simulink model "Demo919"  (R2018b)
settings: Solver=ode3  StartTime=0.0  StopTime=10  FixedStep=0.0005  RelTol=1e-3  EnableMultiTasking=on
values from neighbouring files (symbols this model uses):
  ADS1 = [1000 4000]    [data_new1.m]
  ADS2 = [900 4100]    [data_new1.m]
  br_opening = [0 20 40 60 80 100]    [data_new1.m]
  BRAKE = [485 1288 2091 2894 3697 4500]    [data_new1.m]
  InerWheel_Angle = [0 0.001 0.502 1.006 1.514 2.024 2.538 3.055 3.575 4.098 4.625 5.155 5.689 6.226 6.767 7.311 7.859 8.411 8.967 9.527 10.091 10.659 11.231 11.807 12.387 12.972 13.561 14.154 14.752 15.354 15.961 16.572 17.187 17.807 18.432 19.062 19.696 20.334 20.977 21.625 22.277 22.934 23.596 24.262 24.932 25.607 26.286 26.970 27.657 28.349 29.045 29.745 30.448 31.155 31.866]    [data_new1.m]
  OuterWheel_Angle = [0 0.001 0.501 1.001 1.501 2.001 2.501	3.001 3.501	4.001 4.501	5.001 5.501	6.001 6.501	7.001 7.501	8.001 8.501	9.001 9.501	10.001 10.501 11.001 11.501 12.001 12.501 13.001 13.501	14.001 14.501 15.001 15.501 16.001 16.501 17.001 17.501 18.001 18.501 19.001 19.501	20.001 20.501 21.001 21.501	22.001 22.501 23.001 23.501	24.001 24.501 25.001 25.501 26.001 26.501]    [data_new1.m]
  PUMP = [0 1000 2000 3000 4000 5000]    [data_new1.m]
  SteeringAngle_Cal = [-90 0 90]    [data_new1.m]
  SteeringAngle_Sensor = [640 1840 3041]    [data_new1.m]
  th_opening = [0 100]    [data_new1.m]
undefined symbols (not defined in the file or in its folder): D, I_AN06_5V, I_AN08_5V, I_AN09_5V, I_AN10_5V, I_HALL1, I_HALL2, I_SW01_L, I_SW10_L, I_SW11_H, I_SW12_H, I_SW13_H, I_SW14_H, I_SW15_H, I_SW16_H, I_SW17_H, I_SW18_H, I_SW19_H, I_SW20_H, O_PWM1_LS0A7, O_PWM2_LS0A7, O_SW02_LS0A4, O_SW13_HS1A, O_SW14_HS1A
libraries: ec5744lib x137, simulink x20, canmsglib x11
(part 3 of 5)

== system Demo919/Function-Call Subsystem1/Torque_Control/differential1 ==
  note: 转向半径计算模块
  note: 内外电机转速
  note: 转速差分配
  Steering_Angle : Inport
  Pedal_tr : Inport  Port=2
  MODE : Inport  Port=3
  Abs : Abs
  Add : Sum
  Constant1 : Constant  Value=10000
  Data Type Conversion : DataTypeConversion  OutDataTypeStr=double
  Data Type Conversion3 : DataTypeConversion  OutDataTypeStr=uint16
  Data Type Conversion4 : DataTypeConversion  OutDataTypeStr=uint16
  Gain3 : Gain  Gain=50
  Gain4 : Gain  Gain=2
  MeaModule1 : ec5744lib/RapidECU_U3/07Calibration/MeaModule  signal=InerMotor_RPM
      settings: SourceProductName=ECUCoder for MPC5744
  MeaModule3 : ec5744lib/RapidECU_U3/07Calibration/MeaModule  signal=OuterMotor_RPM
      settings: SourceProductName=ECUCoder for MPC5744
  RPM_Cal1 : Subsystem
  "SteeringAngle " : Subsystem
  Switch : Switch  Criteria=u2 > Threshold  Threshold=15
  Switch1 : Switch  Criteria=u2 > Threshold  Threshold=15
  dynamic_allocation : Stateflow chart  TreatAsAtomicUnit=on
  LMot_Speed : Outport
  RMot_Speed : Outport  Port=2
  SteeringAngle : Outport  Port=3
  wires:
  Steering_Angle/1 -> Data Type Conversion/1
  "SteeringAngle "/2(Turning radius) -> RPM_Cal1/3(Turning radius)
  "SteeringAngle "/1(LR_Flg) -> [LR_Flg]
  [LR_Flg] -> dynamic_allocation/1(LR_Flg)
  Data Type Conversion/1 -> "SteeringAngle "/1(sencor_data)
  RPM_Cal1/1(OuterMotor_RPM) -> MeaModule3/1
  RPM_Cal1/2(InerMotor_PRM) -> MeaModule1/1
  MeaModule3/1 -> Data Type Conversion3/1
  MeaModule1/1 -> Data Type Conversion4/1
  Data Type Conversion3/1 -> dynamic_allocation/2(OuterMotor_RPM)
  Data Type Conversion4/1 -> dynamic_allocation/3(InerMotor_RPM)
  MODE/1 -> RPM_Cal1/2("MODE ")
  Add/1 -> Gain4/1
  Pedal_tr/1 -> Gain3/1, RPM_Cal1/1(Pedal_tr)
  Gain4/1 -> Switch/3, Switch1/3
  "SteeringAngle "/3(SteeringAngle) -> Abs/1, SteeringAngle/1
  Gain3/1 -> Add/1
  Abs/1 -> Switch/2, Switch1/2
  Switch1/1 -> RMot_Speed/1
  Switch/1 -> LMot_Speed/1
  dynamic_allocation/1(LMot_Speed) -> Switch/1
  dynamic_allocation/2(RMot_Speed) -> Switch1/1
  Constant1/1 -> Add/2

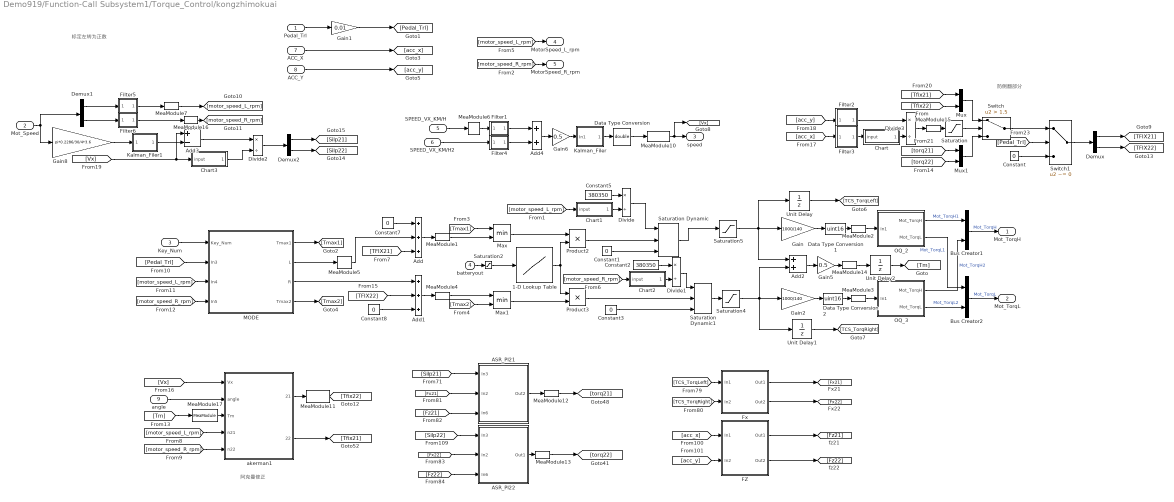
== system Demo919/Function-Call Subsystem1/Torque_Control/kongzhimokuai ==
  note: 阿克曼修正
  note: 防侧翻部分
  note: 标定左转为正数
  Pedal_Trl : Inport
  Mot_Speed : Inport  Port=2
  Key_Num : Inport  Port=3
  batteryout : Inport  Port=4
  SPEED_VX_KM/H : Inport  Port=5
  SPEED_VX_KM/H2 : Inport  Port=6
  ACC_X : Inport  Port=7
  ACC_Y : Inport  Port=8
  angle : Inport  Port=9
  1-D Lookup Table : Lookup_n-D  NumberOfTableDimensions=1  BreakpointsForDimension1=[0 10 20 30 40 50 60 70 72 74 76 78 80 85 100]  Table=[1 1 1 1 1 1 1 1 1 1 0.98 0.97 0.95 0.9 0.5]  InternalRulePriority=Speed  RndMeth=Simplest  InputSameDT=on
  ASR_PI21 : Subsystem
  ASR_PI22 : Subsystem
  Add : Sum  Inputs=+++
  Add1 : Sum  Inputs=+++
  Add2 : Sum
  Add3 : Sum  Inputs=+-
  Add4 : Sum
  Bus Creator1 : BusCreator  Inputs=2
  Bus Creator2 : BusCreator  Inputs=2
  Chart : Stateflow chart  TreatAsAtomicUnit=on
  Chart1 : Stateflow chart  TreatAsAtomicUnit=on
  Chart2 : Stateflow chart  TreatAsAtomicUnit=on
  Chart3 : Stateflow chart  TreatAsAtomicUnit=on
  Constant{,1,3,7..8} (5 alike) : Constant  Value=0
  Constant2 : Constant  Value=380350
  Constant5 : Constant  Value=380350
  Data Type Conversion : DataTypeConversion  OutDataTypeStr=double
  Data Type Conversion1 : DataTypeConversion  OutDataTypeStr=uint16  SaturateOnIntegerOverflow=on
  Data Type Conversion2 : DataTypeConversion  OutDataTypeStr=uint16  SaturateOnIntegerOverflow=on
  Demux : Demux  Outputs=2
  Demux1 : Demux  Outputs=2
  Demux2 : Demux  Outputs=2
  Divide{,1..3} (4 alike) : Product  Inputs=*/
  FZ : Subsystem
  Filter1 : Subsystem
  Filter2 : Subsystem
  Filter3 : Subsystem
  Filter4 : Subsystem
  Filter5 : Subsystem
  Filter6 : Subsystem
  Fx : Subsystem
  Gain : Gain  Gain=1000/140  OutDataTypeStr=double  SaturateOnIntegerOverflow=on
  Gain1 : Gain  Gain=0.01  OutDataTypeStr=double
  Gain2 : Gain  Gain=1000/140  OutDataTypeStr=double  SaturateOnIntegerOverflow=on
  Gain5 : Gain  Gain=0.5  OutDataTypeStr=double
  Gain6 : Gain  Gain=0.5  ParamDataTypeStr=single
  Gain8 : Gain  Gain=pi*0.2286/30/4*3.6
  Kalman_Filer : Subsystem
  Kalman_Filer1 : Subsystem
  MODE : Subsystem
  Max : MinMax  Inputs=2
  Max1 : MinMax  Inputs=2
  MeaModule1 : ec5744lib/RapidECU_U3/07Calibration/MeaModule  signal=c1
      settings: SourceProductName=ECUCoder for MPC5744
  MeaModule10 : ec5744lib/RapidECU_U3/07Calibration/MeaModule  signal=Speed
      settings: SourceProductName=ECUCoder for MPC5744
  MeaModule11 : ec5744lib/RapidECU_U3/07Calibration/MeaModule  signal=b9
      settings: SourceProductName=ECUCoder for MPC5744
  MeaModule12 : ec5744lib/RapidECU_U3/07Calibration/MeaModule  signal=c4
      settings: SourceProductName=ECUCoder for MPC5744
  MeaModule13 : ec5744lib/RapidECU_U3/07Calibration/MeaModule  signal=c5
      settings: SourceProductName=ECUCoder for MPC5744
  MeaModule14 : ec5744lib/RapidECU_U3/07Calibration/MeaModule  signal=c42
      settings: SourceProductName=ECUCoder for MPC5744
  MeaModule15 : ec5744lib/RapidECU_U3/07Calibration/MeaModule  signal=K
      settings: SourceProductName=ECUCoder for MPC5744
  MeaModule16 : ec5744lib/RapidECU_U3/07Calibration/MeaModule  signal=speed22
      settings: SourceProductName=ECUCoder for MPC5744
  MeaModule17 : ec5744lib/RapidECU_U3/07Calibration/MeaModule  signal=b7
      settings: SourceProductName=ECUCoder for MPC5744
  MeaModule2 : ec5744lib/RapidECU_U3/07Calibration/MeaModule  signal=C1
      settings: SourceProductName=ECUCoder for MPC5744
  MeaModule3 : ec5744lib/RapidECU_U3/07Calibration/MeaModule  signal=C2
      settings: SourceProductName=ECUCoder for MPC5744
  MeaModule4 : ec5744lib/RapidECU_U3/07Calibration/MeaModule  signal=c2
      settings: SourceProductName=ECUCoder for MPC5744
  MeaModule5 : ec5744lib/RapidECU_U3/07Calibration/MeaModule  signal=e1
      settings: SourceProductName=ECUCoder for MPC5744
  MeaModule6 : ec5744lib/RapidECU_U3/07Calibration/MeaModule  signal=S11
      settings: SourceProductName=ECUCoder for MPC5744
  MeaModule7 : ec5744lib/RapidECU_U3/07Calibration/MeaModule  signal=speed21
      settings: SourceProductName=ECUCoder for MPC5744
  Mux : Mux  Inputs=2
  Mux1 : Mux  Inputs=2
  OQ_2 : Subsystem
  OQ_3 : Subsystem
  Product2 : Product
  Product3 : Product
  Saturation : Saturate  UpperLimit=2.5  LowerLimit=-2.5
  Saturation Dynamic : simulink/Discontinuities/Saturation Dynamic  OutMin=[]  OutMax=[]  OutDataTypeStr=Inherit: Same as second input  OutDataType=fixdt(1, 16)  OutScaling=2^-10  DoSatur=on
  Saturation Dynamic1 : simulink/Discontinuities/Saturation Dynamic  OutMin=[]  OutMax=[]  OutDataTypeStr=Inherit: Same as second input  OutDataType=fixdt(1, 16)  OutScaling=2^-10  DoSatur=on
  Saturation2 : Saturate  UpperLimit=100  LowerLimit=0
  Saturation4 : Saturate  UpperLimit=140  LowerLimit=0
  Saturation5 : Saturate  UpperLimit=140  LowerLimit=0
  Switch : Switch  Criteria=u2 > Threshold  Threshold=1.5
  Switch1 : Switch  Criteria=u2 ~= 0
  Unit Delay : UnitDelay  SampleTime=-1
  Unit Delay1 : UnitDelay  SampleTime=-1
  Unit Delay2 : UnitDelay  SampleTime=-1
  akerman1 : Subsystem
  Mot_TorqH : Outport
  Mot_TorqL : Outport  Port=2
  speed : Outport  Port=3
  MotorSpeed_L_rpm : Outport  Port=4
  MotorSpeed_R_rpm : Outport  Port=5
  wires:
  [motor_speed_L_rpm] -> MotorSpeed_L_rpm/1
  [motor_speed_R_rpm] -> MotorSpeed_R_rpm/1
  Filter1/1(Out1) -> Add4/1
  Constant/1 -> Switch1/3
  Constant2/1 -> Divide1/1
  [TCS_TorqLeft] -> Fx/1(In1)
  [Vx] -> Chart3/1(input), Add3/1
  MeaModule2/1 -> OQ_2/1(In1)
  Unit Delay2/1 -> [Tm]
  Saturation/1 -> Switch/2
  Add3/1 -> Divide2/1
  Fx/1(Out1) -> [Fx21]
  Chart/1(output) -> Divide3/2
  MODE/1(Tmax1) -> [Tmax1]
  ACC_X/1 -> [acc_x]
  ASR_PI22/1(Out1) -> MeaModule13/1
  MODE/2(L) -> MeaModule5/1
  MeaModule12/1 -> [torq21]
  MeaModule14/1 -> Unit Delay2/1
  MODE/3(R) -> Add1/1
  FZ/1(Out1) -> [Fz21]
  [Silp22] -> ASR_PI22/1(In3)
  Kalman_Filer/1(Out1) -> Data Type Conversion/1
  Data Type Conversion1/1 -> MeaModule2/1
  Demux2/1 -> [Silp21]
  SPEED_VX_KM/H2/1 -> Filter4/1(In1)
  Demux/1 -> [TFIX21]
  Chart3/1(output) -> Divide2/2
  Gain6/1 -> Kalman_Filer/1(In1)
  Add/1 -> MeaModule1/1
  [Tfix22] -> Mux/2
  MeaModule15/1 -> Saturation/1
  [acc_y] -> FZ/2(In2)
  Add4/1 -> Gain6/1
  [Fx21] -> ASR_PI21/2(In2)
  Filter2/1(Out1) -> Divide3/1
  Unit Delay1/1 -> [TCS_TorqRight]
  Pedal_Trl/1 -> Gain1/1
  [acc_y] -> Filter2/1(In1)
  Constant1/1 -> Saturation Dynamic/3
  Filter3/1(Out1) -> Chart/1(input)
  Unit Delay/1 -> [TCS_TorqLeft]
  [motor_speed_L_rpm] -> Chart1/1(input)
  Bus Creator1/1 -> Mot_TorqH/1  "Mot_TorqH"
  MeaModule13/1 -> [torq22]
  Divide/1 -> Saturation Dynamic/1
  Demux2/2 -> [Silp22]
  FZ/2(Out2) -> [Fz22]
  Demux1/2 -> Filter6/1(In1)
  [motor_speed_L_rpm] -> MODE/3(In4)
  [Fz21] -> ASR_PI21/3(In6)
  [acc_x] -> Filter3/1(In1)
  SPEED_VX_KM/H/1 -> MeaModule6/1
  [motor_speed_R_rpm] -> Chart2/1(input)
  Demux/2 -> [TFIX22]
  Gain8/1 -> Kalman_Filer1/1(In1)
  Demux1/1 -> Filter5/1(In1)
  Mux/1 -> Switch/1
  Data Type Conversion2/1 -> MeaModule3/1
  OQ_2/1(Mot_TorqH) -> Bus Creator1/1  "Mot_TorqH1"
  [Fx22] -> ASR_PI22/2(In2)
  [Fz22] -> ASR_PI22/3(In6)
  Mux1/1 -> Switch/3
  [motor_speed_R_rpm] -> MODE/4(In5)
  Divide3/1 -> MeaModule15/1
  Add1/1 -> MeaModule4/1
  MODE/4(Tmax2) -> [Tmax2]
  [acc_x] -> FZ/1(In1)
  Divide2/1 -> Demux2/1
  Fx/2(Out2) -> [Fx22]
  Chart2/1(output) -> Divide1/2
  Chart1/1(output) -> Divide/2
  [TCS_TorqRight] -> Fx/2(In2)
  OQ_3/2(Mot_TorqL) -> Bus Creator2/2  "Mot_TorqL2"
  ACC_Y/1 -> [acc_y]
  [Pedal_Trl] -> Switch1/2
  [torq21] -> Mux1/1
  batteryout/1 -> Saturation2/1
  Max1/1 -> Product3/2
  [Pedal_Trl] -> MODE/2(In3)
  Add2/1 -> Gain5/1
  Switch/1 -> Switch1/1
  Divide1/1 -> Saturation Dynamic1/1
  Filter4/1(Out1) -> Add4/2
  Constant5/1 -> Divide/1
  [Silp21] -> ASR_PI21/1(In3)
  Key_Num/1 -> MODE/1(Key_Num)
  ASR_PI21/1(Out2) -> MeaModule12/1
  OQ_2/2(Mot_TorqL) -> Bus Creator2/1  "Mot_TorqL1"
  Bus Creator2/1 -> Mot_TorqL/1  "Mot_TorqL"
  Gain2/1 -> Data Type Conversion2/1
  Gain/1 -> Data Type Conversion1/1
  MeaModule3/1 -> OQ_3/1(In1)
  Max/1 -> Product2/1
  Gain5/1 -> MeaModule14/1
  [torq22] -> Mux1/2
  OQ_3/1(Mot_TorqH) -> Bus Creator1/2  "Mot_TorqH2"
  [Tfix21] -> Mux/1
  Switch1/1 -> Demux/1
  MeaModule5/1 -> Add/2
  Mot_Speed/1 -> Demux1/1, Gain8/1
  Gain1/1 -> [Pedal_Trl]
  [Tmax1] -> Max/1
  [Tmax2] -> Max1/2
  Data Type Conversion/1 -> MeaModule10/1
  MeaModule6/1 -> Filter1/1(In1)
  Kalman_Filer1/1(Out1) -> Add3/2
  Saturation2/1 -> 1-D Lookup Table/1
  MeaModule10/1 -> [Vx], speed/1
  Constant8/1 -> Add1/3
  Constant7/1 -> Add/1
  1-D Lookup Table/1 -> Product2/2, Product3/1
  Filter5/1(Out1) -> MeaModule7/1
  Filter6/1(Out1) -> MeaModule16/1
  MeaModule7/1 -> [motor_speed_L_rpm]
  MeaModule16/1 -> [motor_speed_R_rpm]
  Product2/1 -> Saturation Dynamic/2
  Saturation Dynamic/1 -> Saturation5/1
  Product3/1 -> Saturation Dynamic1/2
  Constant3/1 -> Saturation Dynamic1/3
  Saturation Dynamic1/1 -> Saturation4/1
  MeaModule11/1 -> [Tfix22]
  [motor_speed_R_rpm] -> akerman1/5(n22)
  angle/1 -> akerman1/2(angle)
  [Vx] -> akerman1/1("Vx ")
  akerman1/2("22 ") -> [Tfix21]
  MeaModule17/1 -> akerman1/3("Tm ")
  [Tm] -> MeaModule17/1
  [motor_speed_L_rpm] -> akerman1/4(n21)
  akerman1/1(21) -> MeaModule11/1
  [TFIX21] -> Add/3
  [TFIX22] -> Add1/2
  MeaModule1/1 -> Max/2
  MeaModule4/1 -> Max1/1
  Saturation5/1 -> Add2/1, Unit Delay/1, Gain/1
  Saturation4/1 -> Add2/2, Gain2/1, Unit Delay1/1

== system Demo919/Function-Call Subsystem1/Torque_Control/Subsystem1/Subsystem ==
  Pedal_WS1 : Inport
  Pedal_Ws2 : Inport  Port=2
  Pedal_Tr : Inport  Port=3
  Constant3 : Constant  Value=0  OutDataTypeStr=uint8
  Logical Operator : Logic  Operator=OR  AllPortsSameDT=off  OutDataTypeStr=boolean
  MeaModule9 : ec5744lib/RapidECU_U3/07Calibration/MeaModule  signal=Pedal_WrongState
      settings: SourceProductName=ECUCoder for MPC5744
  Pedal_Wo_Ar : Switch  Criteria=u2 > Threshold  OutDataTypeStr=double
  Out1 : Outport
  Pedal_WS : Outport  Port=2
  wires:
  MeaModule9/1 -> Pedal_Wo_Ar/2
  Pedal_Ws2/1 -> Logical Operator/2
  Constant3/1 -> Pedal_Wo_Ar/1
  Logical Operator/1 -> Pedal_WS/1, MeaModule9/1
  Pedal_WS1/1 -> Logical Operator/1
  Pedal_Tr/1 -> Pedal_Wo_Ar/3
  Pedal_Wo_Ar/1 -> Out1/1

== system Demo919/Function-Call Subsystem1/Torque_Control/differential1/RPM_Cal1 ==
  note: 计算期望转速和实际转速的误差输入pid，逐渐靠近期望
      | 在两个输出之后新增转速反馈pid
  note: 决定内外轮的速度差异
  note: 内外侧电机期望转速
  Pedal_tr : Inport
  "MODE " : Inport  Port=2
  Turning radius : Inport  Port=3
  Data Type Conversion : DataTypeConversion  OutDataTypeStr=double
  Divide2 : Product  Inputs=*/
  Divide3 : Product  Inputs=*/
  Divide6 : Product  Inputs=**
  Gain1 : Gain  Gain=60
  Gain2 : Gain  Gain=60
  Gain3 : Gain  Gain=4  OutDataTypeStr=double
  Gain4 : Gain  Gain=4  OutDataTypeStr=double
  Gain6 : Gain  Gain=1/100
  Gain7 : Gain  Gain=10/36
  Subsystem : Subsystem
  Tire_perimeter : Subsystem
  Tire_perimeter1 : Subsystem
  dynamic_allocation1 : Stateflow chart  TreatAsAtomicUnit=on
  OuterMotor_RPM : Outport  OutDataTypeStr=double
  InerMotor_PRM : Outport  Port=2  OutDataTypeStr=double
  wires:
  Divide2/1 -> Gain3/1
  Gain1/1 -> Divide2/1
  Gain2/1 -> Divide3/1
  Pedal_tr/1 -> Gain6/1
  Tire_perimeter1/1(D) -> Divide3/2
  Gain3/1 -> OuterMotor_RPM/1
  Divide3/1 -> Gain4/1
  Tire_perimeter/1(D) -> Divide2/2
  Gain4/1 -> InerMotor_PRM/1
  "MODE "/1 -> dynamic_allocation1/1(MODE)
  dynamic_allocation1/1(MAX_SPEED) -> Data Type Conversion/1
  Divide6/1 -> Subsystem/1(set_speed)
  Gain6/1 -> Divide6/2
  Gain7/1 -> Divide6/1
  Turning radius/1 -> Subsystem/2(Turning radius)
  Subsystem/1(Outer_speed) -> Gain1/1
  Subsystem/2(Iner_Speed) -> Gain2/1
  Data Type Conversion/1 -> Gain7/1

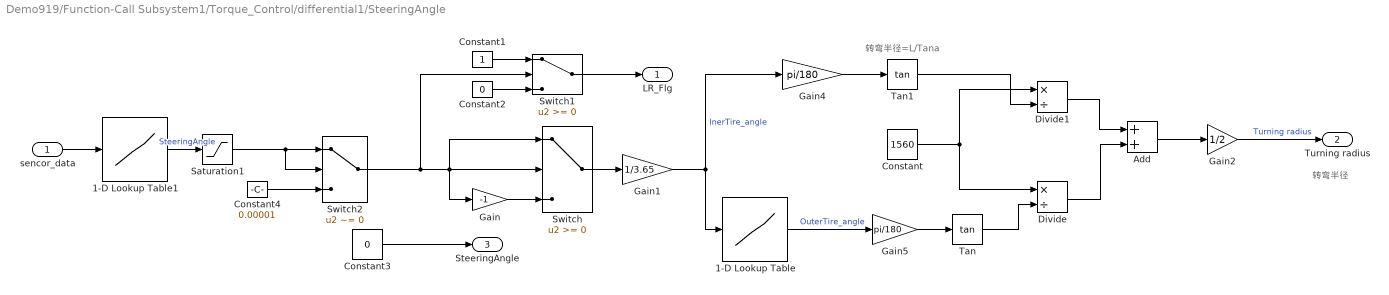
== system Demo919/Function-Call Subsystem1/Torque_Control/differential1/SteeringAngle  ==
  note: 转弯半径=L/Tana
  note: 转弯半径
  sencor_data : Inport
  1-D Lookup Table : Lookup_n-D  NumberOfTableDimensions=1  BreakpointsForDimension1=InerWheel_Angle  Table=OuterWheel_Angle  InternalRulePriority=Speed  RndMeth=Simplest  InputSameDT=on
  1-D Lookup Table1 : Lookup_n-D  NumberOfTableDimensions=1  BreakpointsForDimension1=SteeringAngle_Sensor  Table=SteeringAngle_Cal  InternalRulePriority=Speed  RndMeth=Simplest  InputSameDT=on
  Add : Sum
  Constant : Constant  Value=1560
  Constant1 : Constant
  Constant2 : Constant  Value=0
  Constant3 : Constant  Value=0
  Constant4 : Constant  Value=0.00001
  Divide : Product  Inputs=*/
  Divide1 : Product  Inputs=*/
  Gain : Gain  Gain=-1
  Gain1 : Gain  Gain=1/3.65
  Gain2 : Gain  Gain=1/2
  Gain4 : Gain  Gain=pi/180
  Gain5 : Gain  Gain=pi/180
  Saturation1 : Saturate  UpperLimit=90  LowerLimit=-90
  Switch : Switch
  Switch1 : Switch
  Switch2 : Switch  Criteria=u2 ~= 0
  Tan : Trigonometry  Operator=tan
  Tan1 : Trigonometry  Operator=tan
  LR_Flg : Outport
  Turning radius : Outport  Port=2
  SteeringAngle : Outport  Port=3
  wires:
  Gain1/1 -> Gain4/1, 1-D Lookup Table/1  "InerTire_angle"
  1-D Lookup Table/1 -> Gain5/1  "OuterTire_angle"
  1-D Lookup Table1/1 -> Saturation1/1  "SteeringAngle"
  Add/1 -> Gain2/1
  Divide/1 -> Add/2
  Gain/1 -> Switch/3
  Constant/1 -> Divide1/1, Divide/1
  Switch/1 -> Gain1/1
  Gain2/1 -> Turning radius/1  "Turning radius"
  Tan1/1 -> Divide1/2
  Tan/1 -> Divide/2
  Divide1/1 -> Add/1
  sencor_data/1 -> 1-D Lookup Table1/1
  Gain4/1 -> Tan1/1
  Gain5/1 -> Tan/1
  Constant1/1 -> Switch1/1
  Constant2/1 -> Switch1/3
  Switch1/1 -> LR_Flg/1
  Saturation1/1 -> Switch2/2, Switch2/1
  Constant4/1 -> Switch2/3
  Switch2/1 -> Switch/2, Switch/1, Gain/1, Switch1/2
  Constant3/1 -> SteeringAngle/1

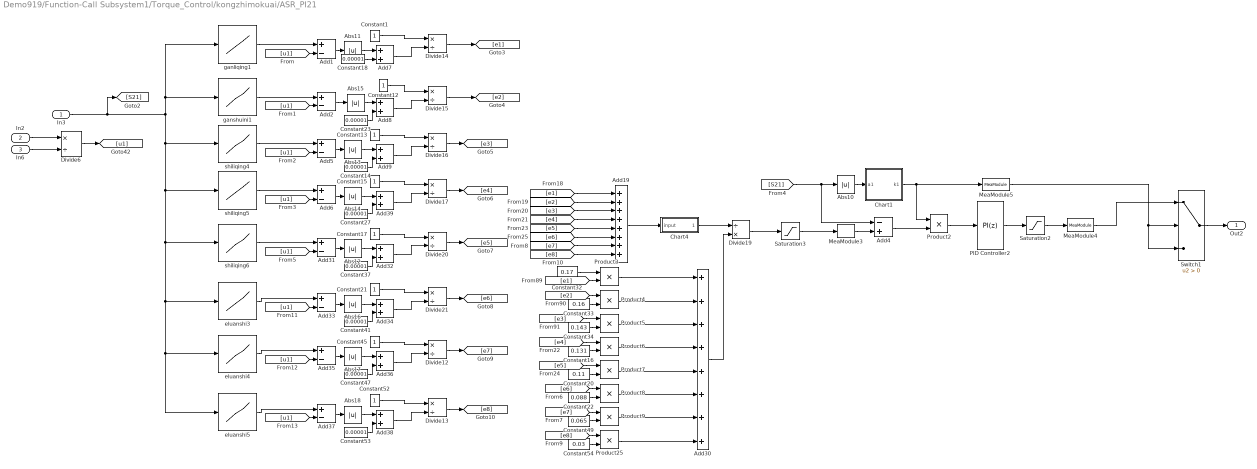
== system Demo919/Function-Call Subsystem1/Torque_Control/kongzhimokuai/ASR_PI21 ==
  In3 : Inport
  In2 : Inport  Port=2
  In6 : Inport  Port=3
  Abs{10..18} (9 alike) : Abs
  Add{1..2,5..6,31,33,35,37} (8 alike) : Sum  Inputs=+-
  Add19 : Sum  Inputs=++++++++
  Add30 : Sum  Inputs=++++++++
  Add{7..9,32,34,36,38..39} (8 alike) : Sum
  Add4 : Sum  Inputs=-+
  Chart1 : Stateflow chart  TreatAsAtomicUnit=on
  Chart4 : Stateflow chart  TreatAsAtomicUnit=on
  Constant{1,12..13,15,17,21,45,52} (8 alike) : Constant
  Constant{14,18,23,27,37,41,47,53} (8 alike) : Constant  Value=0.00001
  Constant16 : Constant  Value=0.131
  Constant20 : Constant  Value=0.11
  Constant22 : Constant  Value=0.088
  Constant32 : Constant  Value=0.17
  Constant33 : Constant  Value=0.16
  Constant34 : Constant  Value=0.143
  Constant49 : Constant  Value=0.065
  Constant54 : Constant  Value=0.03
  Divide{6,12..17,20..21} (9 alike) : Product  Inputs=*/
  Divide19 : Product  Inputs=/*
  MeaModule3 : ec5744lib/RapidECU_U3/07Calibration/MeaModule  signal=s_t
      settings: SourceProductName=ECUCoder for MPC5744
  MeaModule4 : ec5744lib/RapidECU_U3/07Calibration/MeaModule  signal=S_21
      settings: SourceProductName=ECUCoder for MPC5744
  MeaModule5 : ec5744lib/RapidECU_U3/07Calibration/MeaModule  signal=S_211
      settings: SourceProductName=ECUCoder for MPC5744
  PID Controller2 : simulink/Continuous/PID Controller  Controller=PI  Form=Parallel  TimeDomain=Discrete-time  SampleTime=-1  IntegratorMethod=Forward Euler  FilterMethod=Forward Euler  ControllerParametersSource=internal  P=156  I=25  D=D  UseFilter=on  N=100  TunerSelectOption=Transfer Function Based (PID Tuner App)  InitialConditionSource=internal  InitialConditionForIntegrator=0  InitialConditionForFilter=0  DifferentiatorICPrevScaledInput=0  ExternalReset=none  TrackingMode=off  Kt=1  LimitOutput=on  UpperSaturationLimit=inf  LowerSaturationLimit=-inf  LinearizeAsGain=on  AntiWindupMode=clamping  Kb=1  POutMin=[]  POutMax=[]  IOutMin=[]  IOutMax=[]  DOutMin=[]  DOutMax=[]  NOutMin=[]  NOutMax=[]  SumOutMin=[]  SumOutMax=[]  SaturationOutMin=[]  SaturationOutMax=[]  PParamMin=[]  PParamMax=[]  IParamMin=[]  IParamMax=[]  DParamMin=[]  DParamMax=[]  NParamMin=[]  NParamMax=[]  KbParamMin=[]  KbParamMax=[]  KtParamMin=[]  KtParamMax=[]  KbOutMin=[]  KbOutMax=[]  KtOutMin=[]  KtOutMax=[]  IntegratorOutMin=[]  IntegratorOutMax=[]  FilterOutMin=[]  FilterOutMax=[]  SumI1OutMin=[]  SumI1OutMax=[]  SumI2OutMin=[]  SumI2OutMax=[]  SumI3OutMin=[]  SumI3OutMax=[]  SumI4OutMin=[]  SumI4OutMax=[]  SumDOutMin=[]  SumDOutMax=[]  DifferentiatorOutMin=[]  DifferentiatorOutMax=[]  FilterDiffOutCoefMin=[]  FilterDiffOutCoefMax=[]  ReciprocalOutMin=[]  ReciprocalOutMax=[]  SumDenOutMin=[]  SumDenOutMax=[]  SumNumOutMin=[]  SumNumOutMax=[]  DivideOutMin=[]  DivideOutMax=[]  IntegratorContinuousStateAttributes=''  IntegratorStateMustResolveToSignalObject=off  IntegratorRTWStateStorageClass=Auto  FilterContinuousStateAttributes=''  FilterStateMustResolveToSignalObject=off  FilterRTWStateStorageClass=Auto  ParallelPVariant=InternalParameters  IdealPVariant=Disabled  IVariant=InternalParameters  DVariant=Disabled  IntegratorVariant=Discrete  SatVariant=Enabled  AWVariant=DiscClampingParallel  PCopyVariant=Disabled  TRVariant=Disabled  FdbkBlocksVariant=Forward  IdealPFdbkVariant=Disabled  SatFdbkVariant=Disabled  DerivativeFilterVariant=Disabled  NVariant=Disabled  NCopyVariant=Disabled_SignalSpec  FilterICVariant=Disabled  IntegratorICVariant=InternalICs  ExternalResetVariant=Disabled  TRSumVariant=Passthrough  SumFdbkVariant=Disabled  SumVariant=Sum_PI
  Product{2..9,25} (9 alike) : Product
  Saturation2 : Saturate  UpperLimit=15  LowerLimit=-15
  Saturation3 : Saturate  UpperLimit=0.2  LowerLimit=0
  Switch1 : Switch  Criteria=u2 > Threshold
  eluanshi3 : Lookup_n-D  NumberOfTableDimensions=1  BreakpointsForDimension1=[0.00591,0.009,0.01212,0.01856,0.0196,0.02707,0.03557,0.04385,0.05236,0.06524,0.1011,0.13927,0.18595,0.21975,0.26849,0.32574,0.38507,0.44646,0.51635,0.58188,0.63914,0.70697,0.78123,0.86792,0.92103,0.97184,0.993]  Table=[0.04929,0.12757,0.19671,0.25086,0.2838,0.31087,0.34088,0.36501,0.38001,0.38915,0.38915,0.38621,0.38295,0.37414,0.37121,0.36208,0.35588,0.34707,0.33794,0.335,0.32587,0.31707,0.31087,0.2988,0.29293,0.28673,0.2838]  InternalRulePriority=Speed  RndMeth=Simplest  InputSameDT=on
  eluanshi4 : Lookup_n-D  NumberOfTableDimensions=1  BreakpointsForDimension1=|  Table=|  InternalRulePriority=Speed  RndMeth=Simplest  InputSameDT=on
      BreakpointsForDimension1=|
      | [0.00154
      | 0.00798
      | 0.01649
      | 0.0227
      | 0.03121
      | 0.04178
      | 0.05673
      | 0.12433
      | 0.19216
      | 0.26642
      | 0.36598
      | 0.4952
      | 0.61591
      | 0.79388
      | 0.91873
      | 1.00357]
      Table=|
      | [0.04636
      | 0.11257
      | 0.14257
      | 0.17551
      | 0.18465
      | 0.19052
      | 0.19052
      | 0.18758
      | 0.18465
      | 0.17551
      | 0.17258
      | 0.16051
      | 0.15758
      | 0.14551
      | 0.13638
      | 0.1305]
  eluanshi5 : Lookup_n-D  NumberOfTableDimensions=1  BreakpointsForDimension1=|  Table=|  InternalRulePriority=Speed  RndMeth=Simplest  InputSameDT=on
      BreakpointsForDimension1=|
      | [0.00361
      | 0.00798
      | 0.01212
      | 0.01419
      | 0.01856
      | 0.0227
      | 0.02707
      | 0.02914
      | 0.04178
      | 0.09903
      | 0.15836
      | 0.26435
      | 0.37012
      | 0.49934
      | 0.60327
      | 0.69225
      | 0.78537
      | 0.86792
      | 0.94425
      | 1.0015]
      Table=|
      | [0.05549
      | 0.1093
      | 0.13964
      | 0.1517
      | 0.16051
      | 0.16964
      | 0.17845
      | 0.18465
      | 0.19052
      | 0.19052
      | 0.18465
      | 0.17845
      | 0.17258
      | 0.16671
      | 0.15758
      | 0.15464
      | 0.14551
      | 0.14257
      | 0.13638
      | 0.13344]
  ganliqing1 : Lookup_n-D  NumberOfTableDimensions=1  BreakpointsForDimension1=|  Table=|  InternalRulePriority=Speed  RndMeth=Simplest  InputSameDT=on
      BreakpointsForDimension1=|
      | [0.01498
      | 0.03128
      | 0.05446
      | 0.06846
      | 0.08017
      | 0.09165
      | 0.10335
      | 0.11506
      | 0.12424
      | 0.13595
      | 0.15454
      | 0.16625
      | 0.17772
      | 0.19632
      | 0.22202
      | 0.25691
      | 0.31499
      | 0.38017
      | 0.49196
      | 0.59433
      | 0.70129
      | 0.80367
      | 0.86885
      | 0.95493
      | 0.999]
      Table=|
      | [0.38854
      | 0.66554
      | 0.92268
      | 1.00503
      | 1.04474
      | 1.08738
      | 1.12058
      | 1.13686
      | 1.1502
      | 1.16322
      | 1.1668
      | 1.1668
      | 1.1668
      | 1.16322
      | 1.15346
      | 1.14044
      | 1.11049
      | 1.07762
      | 1.02489
      | 0.9689
      | 0.91617
      | 0.86019
      | 0.82699
      | 0.78435
      | 0.76123]
  ganshuini1 : Lookup_n-D  NumberOfTableDimensions=1  BreakpointsForDimension1=|  Table=|  InternalRulePriority=Speed  RndMeth=Simplest  InputSameDT=on
      BreakpointsForDimension1=|
      | [0
      | 0.00612
      | 0.01323
      | 0.0185
      | 0.024
      | 0.03293
      | 0.04531
      | 0.05241
      | 0.06295
      | 0.06845
      | 0.07555
      | 0.08266
      | 0.08976
      | 0.0932
      | 0.10213
      | 0.11107
      | 0.12161
      | 0.13055
      | 0.14315
      | 0.15369
      | 0.17156
      | 0.18577
      | 0.19631
      | 0.21419
      | 0.2355
      | 0.25497
      | 0.27468
      | 0.28889
      | 0.30676
      | 0.3173
      | 0.33334
      | 0.35465
      | 0.37252
      | 0.3991
      | 0.41858
      | 0.44539
      | 0.46143
      | 0.48985
      | 0.51299
      | 0.53613
      | 0.55194
      | 0.56798
      | 0.59823
      | 0.6161
      | 0.64085
      | 0.66926
      | 0.69424
      | 0.69791
      | 0.71211
      | 0.75107
      | 0.79209
      | 0.81706
      | 0.85075
      | 0.89887
      | 0.93599
      | 0.98411
      | 0.99832]
      Table=|
      | [0.0357
      | 0.13134
      | 0.30251
      | 0.41079
      | 0.52393
      | 0.63999
      | 0.78847
      | 0.84617
      | 0.90679
      | 0.9444
      | 0.97228
      | 0.99238
      | 1.01248
      | 1.02512
      | 1.04263
      | 1.05787
      | 1.06532
      | 1.07537
      | 1.07797
      | 1.08056
      | 1.08056
      | 1.07797
      | 1.07537
      | 1.06792
      | 1.05527
      | 1.05009
      | 1.04004
      | 1.03258
      | 1.02512
      | 1.01994
      | 1.00989
      | 0.99724
      | 0.98979
      | 0.97455
      | 0.9645
      | 0.94959
      | 0.94181
      | 0.92949
      | 0.91425
      | 0.90161
      | 0.89156
      | 0.8841
      | 0.86886
      | 0.86141
      | 0.84876
      | 0.82867
      | 0.81602
      | 0.81343
      | 0.80857
      | 0.78587
      | 0.76318
      | 0.75313
      | 0.73562
      | 0.70547
      | 0.69024
      | 0.66268
      | 0.6549]
  shiliqing4 : Lookup_n-D  NumberOfTableDimensions=1  BreakpointsForDimension1=|  Table=|  InternalRulePriority=Speed  RndMeth=Simplest  InputSameDT=on
      BreakpointsForDimension1=|
      | [0.00269
      | 0.00429
      | 0.01139
      | 0.01689
      | 0.02033
      | 0.0256
      | 0.0311
      | 0.04004
      | 0.04874
      | 0.06135
      | 0.07372
      | 0.08609
      | 0.0987
      | 0.11451
      | 0.13948
      | 0.1734
      | 0.20342
      | 0.23023
      | 0.24787
      | 0.26391
      | 0.28522
      | 0.30676
      | 0.3173
      | 0.35465
      | 0.39383
      | 0.42935
      | 0.47564
      | 0.51826
      | 0.55905
      | 0.59113
      | 0.63925
      | 0.68003
      | 0.72266
      | 0.7529
      | 0.79552
      | 0.84548
      | 0.89153
      | 0.92545
      | 0.99488]
      Table=|
      | [0.04835
      | 0.16927
      | 0.24707
      | 0.3278
      | 0.39328
      | 0.54662
      | 0.63221
      | 0.70547
      | 0.76059
      | 0.82607
      | 0.87405
      | 0.89901
      | 0.9243
      | 0.93694
      | 0.93954
      | 0.93694
      | 0.92689
      | 0.92171
      | 0.90906
      | 0.9042
      | 0.89415
      | 0.8841
      | 0.87665
      | 0.864
      | 0.84876
      | 0.82867
      | 0.81116
      | 0.79592
      | 0.77323
      | 0.75832
      | 0.74049
      | 0.72298
      | 0.70029
      | 0.69024
      | 0.67014
      | 0.64744
      | 0.62994
      | 0.6147
      | 0.58196]
  shiliqing5 : Lookup_n-D  NumberOfTableDimensions=1  BreakpointsForDimension1=|  Table=|  InternalRulePriority=Speed  RndMeth=Simplest  InputSameDT=on
      BreakpointsForDimension1=|
      | [8.52288E-4
      | 0.00429
      | 0.00612
      | 0.00796
      | 0.01139
      | 0.01506
      | 0.01689
      | 0.0185
      | 0.02033
      | 0.02216
      | 0.0256
      | 0.02927
      | 0.03454
      | 0.0382
      | 0.04164
      | 0.04714
      | 0.05058
      | 0.05768
      | 0.06478
      | 0.07189
      | 0.08082
      | 0.08793
      | 0.0932
      | 0.0987
      | 0.1058
      | 0.1129
      | 0.12528
      | 0.14315
      | 0.1876
      | 0.21052
      | 0.23023
      | 0.25337
      | 0.29072
      | 0.33678
      | 0.40437
      | 0.48435
      | 0.55561
      | 0.6035
      | 0.70662
      | 0.76894
      | 0.84364
      | 0.92018
      | 1.00015]
      Table=|
      | [0.04575
      | 0.09859
      | 0.14139
      | 0.19423
      | 0.24221
      | 0.285
      | 0.33525
      | 0.37059
      | 0.40074
      | 0.43348
      | 0.46622
      | 0.53171
      | 0.56672
      | 0.59201
      | 0.62475
      | 0.65231
      | 0.675
      | 0.71034
      | 0.73789
      | 0.75313
      | 0.77064
      | 0.77842
      | 0.78328
      | 0.78847
      | 0.79592
      | 0.79852
      | 0.79852
      | 0.79333
      | 0.78587
      | 0.77842
      | 0.77064
      | 0.76577
      | 0.75313
      | 0.73562
      | 0.71293
      | 0.68505
      | 0.66009
      | 0.64485
      | 0.6147
      | 0.58715
      | 0.56186
      | 0.53657
      | 0.50902]
  shiliqing6 : Lookup_n-D  NumberOfTableDimensions=1  BreakpointsForDimension1=|  Table=|  InternalRulePriority=Speed  RndMeth=Simplest  InputSameDT=on
      BreakpointsForDimension1=|
      | [0.0
      | 0.00154
      | 0.00798
      | 0.01212
      | 0.01419
      | 0.01856
      | 0.02477
      | 0.02914
      | 0.03764
      | 0.04615
      | 0.05236
      | 0.05673
      | 0.06087
      | 0.06937
      | 0.07788
      | 0.08846
      | 0.10317
      | 0.11812
      | 0.1372
      | 0.16893
      | 0.20503
      | 0.24941
      | 0.29171
      | 0.32988
      | 0.37012
      | 0.41243
      | 0.45496
      | 0.49083
      | 0.529
      | 0.57775
      | 0.62856
      | 0.68167
      | 0.73249
      | 0.77686
      | 0.82975
      | 0.90608
      | 0.94839
      | 1]
      Table=|
      | [0.0
      | 0.09756
      | 0.14551
      | 0.20878
      | 0.25379
      | 0.32
      | 0.35588
      | 0.39208
      | 0.44329
      | 0.47917
      | 0.50624
      | 0.5245
      | 0.5395
      | 0.55451
      | 0.57245
      | 0.58158
      | 0.59071
      | 0.59952
      | 0.59658
      | 0.59365
      | 0.58745
      | 0.57864
      | 0.57245
      | 0.56364
      | 0.55451
      | 0.54831
      | 0.5395
      | 0.53331
      | 0.5245
      | 0.51537
      | 0.5033
      | 0.49417
      | 0.48536
      | 0.47623
      | 0.46416
      | 0.44916
      | 0.44329
      | 0.43122]
  Out2 : Outport
  wires:
  MeaModule3/1 -> Add4/2
  Add4/1 -> Product2/2
  PID Controller2/1 -> Saturation2/1
  Add19/1 -> Chart4/1(input)
  Constant13/1 -> Divide16/1
  MeaModule4/1 -> Switch1/1
  In2/1 -> Divide6/1
  Divide6/1 -> [u1]
  Chart1/1(k1) -> Product2/1, MeaModule5/1
  [S21] -> Abs10/1, Add4/1
  In3/1 -> [S21], ganliqing1/1, ganshuini1/1, eluanshi4/1, eluanshi5/1, eluanshi3/1, shiliqing6/1, shiliqing5/1, shiliqing4/1
  Add33/1 -> Abs16/1
  Add39/1 -> Divide17/2
  Add35/1 -> Abs17/1
  Constant22/1 -> Product8/2
  eluanshi5/1 -> Add37/1
  [e7] -> Product9/1
  Constant54/1 -> Product25/2
  Constant27/1 -> Add39/2
  Constant21/1 -> Divide21/1
  Constant34/1 -> Product5/2
  Product4/1 -> Add30/2
  Constant33/1 -> Product4/2
  Divide15/1 -> [e2]
  Abs12/1 -> Add32/1
  Constant16/1 -> Product6/2
  Constant47/1 -> Add36/2
  shiliqing4/1 -> Add5/1
  Add37/1 -> Abs18/1
  eluanshi3/1 -> Add33/1
  [e5] -> Add19/5
  [e4] -> Product6/1
  Add8/1 -> Divide15/2
  Constant15/1 -> Divide17/1
  Add9/1 -> Divide16/2
  [e6] -> Product8/1
  Constant23/1 -> Add8/2
  [e1] -> Add19/1
  Add6/1 -> Abs14/1
  [e2] -> Add19/2
  Add7/1 -> Divide14/2
  Constant32/1 -> Product3/1
  Abs15/1 -> Add8/1
  Saturation3/1 -> MeaModule3/1
  [u1] -> Add6/2
  [u1] -> Add31/2
  Abs14/1 -> Add39/1
  Divide13/1 -> [e8]
  [u1] -> Add37/2
  Abs13/1 -> Add9/1
  Abs17/1 -> Add36/1
  Abs18/1 -> Add38/1
  Abs16/1 -> Add34/1
  [e7] -> Add19/7
  Add5/1 -> Abs13/1
  ganshuini1/1 -> Add2/1
  Divide20/1 -> [e5]
  Add38/1 -> Divide13/2
  Divide17/1 -> [e4]
  [u1] -> Add5/2
  Constant45/1 -> Divide12/1
  Add34/1 -> Divide21/2
  [u1] -> Add1/2
  Divide14/1 -> [e1]
  Constant53/1 -> Add38/2
  [e8] -> Product25/1
  Constant17/1 -> Divide20/1
  shiliqing6/1 -> Add31/1
  Product9/1 -> Add30/7
  Divide21/1 -> [e6]
  Product25/1 -> Add30/8
  Add1/1 -> Abs11/1
  [e8] -> Add19/8
  [e3] -> Product5/1
  Product5/1 -> Add30/3
  shiliqing5/1 -> Add6/1
  [e5] -> Product7/1
  [e3] -> Add19/3
  Constant12/1 -> Divide15/1
  Abs10/1 -> Chart1/1(a1)
  Product2/1 -> PID Controller2/1
  Constant14/1 -> Add9/2
  ganliqing1/1 -> Add1/1
  [u1] -> Add33/2
  Saturation2/1 -> MeaModule4/1
  Constant20/1 -> Product7/2
  Add31/1 -> Abs12/1
  Add2/1 -> Abs15/1
  Constant37/1 -> Add32/2
  Switch1/1 -> Out2/1
  Divide19/1 -> Saturation3/1
  [e4] -> Add19/4
  Product8/1 -> Add30/6
  Product3/1 -> Add30/1
  Constant18/1 -> Add7/2
  Add30/1 -> Divide19/2
  Divide16/1 -> [e3]
  [e2] -> Product4/1
  eluanshi4/1 -> Add35/1
  Constant41/1 -> Add34/2
  [e6] -> Add19/6
  [u1] -> Add2/2
  In6/1 -> Divide6/2
  Constant1/1 -> Divide14/1
  Product6/1 -> Add30/4
  [u1] -> Add35/2
  [e1] -> Product3/2
  MeaModule5/1 -> Switch1/3, Switch1/2
  Constant52/1 -> Divide13/1
  Constant49/1 -> Product9/2
  Add32/1 -> Divide20/2
  Divide12/1 -> [e7]
  Chart4/1(output) -> Divide19/1
  Add36/1 -> Divide12/2
  Product7/1 -> Add30/5
  Abs11/1 -> Add7/1

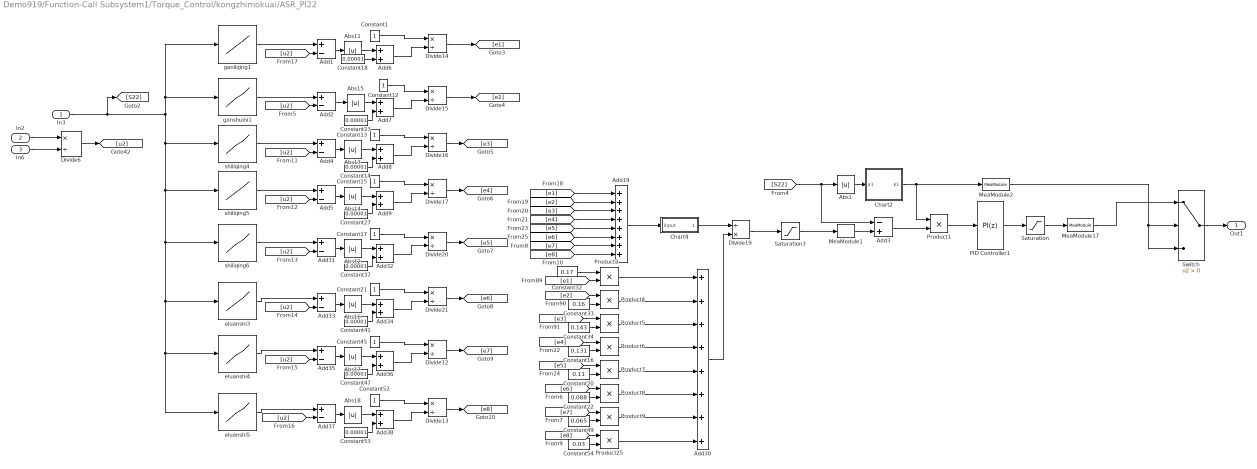
== system Demo919/Function-Call Subsystem1/Torque_Control/kongzhimokuai/ASR_PI22 ==
  In3 : Inport
  In2 : Inport  Port=2
  In6 : Inport  Port=3
  Abs{1,11..18} (9 alike) : Abs
  Add{1..2,4..5,31,33,35,37} (8 alike) : Sum  Inputs=+-
  Add19 : Sum  Inputs=++++++++
  Add3 : Sum  Inputs=-+
  Add30 : Sum  Inputs=++++++++
  Add{6..9,32,34,36,38} (8 alike) : Sum
  Chart2 : Stateflow chart  TreatAsAtomicUnit=on
  Chart4 : Stateflow chart  TreatAsAtomicUnit=on
  Constant{1,12..13,15,17,21,45,52} (8 alike) : Constant
  Constant{14,18,23,27,37,41,47,53} (8 alike) : Constant  Value=0.00001
  Constant16 : Constant  Value=0.131
  Constant20 : Constant  Value=0.11
  Constant22 : Constant  Value=0.088
  Constant32 : Constant  Value=0.17
  Constant33 : Constant  Value=0.16
  Constant34 : Constant  Value=0.143
  Constant49 : Constant  Value=0.065
  Constant54 : Constant  Value=0.03
  Divide{6,12..17,20..21} (9 alike) : Product  Inputs=*/
  Divide19 : Product  Inputs=/*
  MeaModule1 : ec5744lib/RapidECU_U3/07Calibration/MeaModule  signal=s_t7
      settings: SourceProductName=ECUCoder for MPC5744
  MeaModule17 : ec5744lib/RapidECU_U3/07Calibration/MeaModule  signal=S_217
      settings: SourceProductName=ECUCoder for MPC5744
  MeaModule2 : ec5744lib/RapidECU_U3/07Calibration/MeaModule  signal=S_2117
      settings: SourceProductName=ECUCoder for MPC5744
  PID Controller1 : simulink/Continuous/PID Controller  Controller=PI  Form=Parallel  TimeDomain=Discrete-time  SampleTime=-1  IntegratorMethod=Forward Euler  FilterMethod=Forward Euler  ControllerParametersSource=internal  P=156  I=25  D=D  UseFilter=on  N=100  TunerSelectOption=Transfer Function Based (PID Tuner App)  InitialConditionSource=internal  InitialConditionForIntegrator=0  InitialConditionForFilter=0  DifferentiatorICPrevScaledInput=0  ExternalReset=none  TrackingMode=off  Kt=1  LimitOutput=on  UpperSaturationLimit=inf  LowerSaturationLimit=-inf  LinearizeAsGain=on  AntiWindupMode=clamping  Kb=1  POutMin=[]  POutMax=[]  IOutMin=[]  IOutMax=[]  DOutMin=[]  DOutMax=[]  NOutMin=[]  NOutMax=[]  SumOutMin=[]  SumOutMax=[]  SaturationOutMin=[]  SaturationOutMax=[]  PParamMin=[]  PParamMax=[]  IParamMin=[]  IParamMax=[]  DParamMin=[]  DParamMax=[]  NParamMin=[]  NParamMax=[]  KbParamMin=[]  KbParamMax=[]  KtParamMin=[]  KtParamMax=[]  KbOutMin=[]  KbOutMax=[]  KtOutMin=[]  KtOutMax=[]  IntegratorOutMin=[]  IntegratorOutMax=[]  FilterOutMin=[]  FilterOutMax=[]  SumI1OutMin=[]  SumI1OutMax=[]  SumI2OutMin=[]  SumI2OutMax=[]  SumI3OutMin=[]  SumI3OutMax=[]  SumI4OutMin=[]  SumI4OutMax=[]  SumDOutMin=[]  SumDOutMax=[]  DifferentiatorOutMin=[]  DifferentiatorOutMax=[]  FilterDiffOutCoefMin=[]  FilterDiffOutCoefMax=[]  ReciprocalOutMin=[]  ReciprocalOutMax=[]  SumDenOutMin=[]  SumDenOutMax=[]  SumNumOutMin=[]  SumNumOutMax=[]  DivideOutMin=[]  DivideOutMax=[]  IntegratorContinuousStateAttributes=''  IntegratorStateMustResolveToSignalObject=off  IntegratorRTWStateStorageClass=Auto  FilterContinuousStateAttributes=''  FilterStateMustResolveToSignalObject=off  FilterRTWStateStorageClass=Auto  ParallelPVariant=InternalParameters  IdealPVariant=Disabled  IVariant=InternalParameters  DVariant=Disabled  IntegratorVariant=Discrete  SatVariant=Enabled  AWVariant=DiscClampingParallel  PCopyVariant=Disabled  TRVariant=Disabled  FdbkBlocksVariant=Forward  IdealPFdbkVariant=Disabled  SatFdbkVariant=Disabled  DerivativeFilterVariant=Disabled  NVariant=Disabled  NCopyVariant=Disabled_SignalSpec  FilterICVariant=Disabled  IntegratorICVariant=InternalICs  ExternalResetVariant=Disabled  TRSumVariant=Passthrough  SumFdbkVariant=Disabled  SumVariant=Sum_PI
  Product{1,3..9,25} (9 alike) : Product
  Saturation : Saturate  UpperLimit=15  LowerLimit=-15
  Saturation3 : Saturate  UpperLimit=0.2  LowerLimit=0
  Switch : Switch  Criteria=u2 > Threshold
  eluanshi3 : Lookup_n-D  NumberOfTableDimensions=1  BreakpointsForDimension1=[0.00591,0.009,0.01212,0.01856,0.0196,0.02707,0.03557,0.04385,0.05236,0.06524,0.1011,0.13927,0.18595,0.21975,0.26849,0.32574,0.38507,0.44646,0.51635,0.58188,0.63914,0.70697,0.78123,0.86792,0.92103,0.97184,0.993]  Table=[0.04929,0.12757,0.19671,0.25086,0.2838,0.31087,0.34088,0.36501,0.38001,0.38915,0.38915,0.38621,0.38295,0.37414,0.37121,0.36208,0.35588,0.34707,0.33794,0.335,0.32587,0.31707,0.31087,0.2988,0.29293,0.28673,0.2838]  InternalRulePriority=Speed  RndMeth=Simplest  InputSameDT=on
  eluanshi4 : Lookup_n-D  NumberOfTableDimensions=1  BreakpointsForDimension1=|  Table=|  InternalRulePriority=Speed  RndMeth=Simplest  InputSameDT=on
      BreakpointsForDimension1=|
      | [0.00154
      | 0.00798
      | 0.01649
      | 0.0227
      | 0.03121
      | 0.04178
      | 0.05673
      | 0.12433
      | 0.19216
      | 0.26642
      | 0.36598
      | 0.4952
      | 0.61591
      | 0.79388
      | 0.91873
      | 1.00357]
      Table=|
      | [0.04636
      | 0.11257
      | 0.14257
      | 0.17551
      | 0.18465
      | 0.19052
      | 0.19052
      | 0.18758
      | 0.18465
      | 0.17551
      | 0.17258
      | 0.16051
      | 0.15758
      | 0.14551
      | 0.13638
      | 0.1305]
  eluanshi5 : Lookup_n-D  NumberOfTableDimensions=1  BreakpointsForDimension1=|  Table=|  InternalRulePriority=Speed  RndMeth=Simplest  InputSameDT=on
      BreakpointsForDimension1=|
      | [0.00361
      | 0.00798
      | 0.01212
      | 0.01419
      | 0.01856
      | 0.0227
      | 0.02707
      | 0.02914
      | 0.04178
      | 0.09903
      | 0.15836
      | 0.26435
      | 0.37012
      | 0.49934
      | 0.60327
      | 0.69225
      | 0.78537
      | 0.86792
      | 0.94425
      | 1.0015]
      Table=|
      | [0.05549
      | 0.1093
      | 0.13964
      | 0.1517
      | 0.16051
      | 0.16964
      | 0.17845
      | 0.18465
      | 0.19052
      | 0.19052
      | 0.18465
      | 0.17845
      | 0.17258
      | 0.16671
      | 0.15758
      | 0.15464
      | 0.14551
      | 0.14257
      | 0.13638
      | 0.13344]
  ganliqing1 : Lookup_n-D  NumberOfTableDimensions=1  BreakpointsForDimension1=|  Table=|  InternalRulePriority=Speed  RndMeth=Simplest  InputSameDT=on
      BreakpointsForDimension1=|
      | [0.01498
      | 0.03128
      | 0.05446
      | 0.06846
      | 0.08017
      | 0.09165
      | 0.10335
      | 0.11506
      | 0.12424
      | 0.13595
      | 0.15454
      | 0.16625
      | 0.17772
      | 0.19632
      | 0.22202
      | 0.25691
      | 0.31499
      | 0.38017
      | 0.49196
      | 0.59433
      | 0.70129
      | 0.80367
      | 0.86885
      | 0.95493
      | 0.999]
      Table=|
      | [0.38854
      | 0.66554
      | 0.92268
      | 1.00503
      | 1.04474
      | 1.08738
      | 1.12058
      | 1.13686
      | 1.1502
      | 1.16322
      | 1.1668
      | 1.1668
      | 1.1668
      | 1.16322
      | 1.15346
      | 1.14044
      | 1.11049
      | 1.07762
      | 1.02489
      | 0.9689
      | 0.91617
      | 0.86019
      | 0.82699
      | 0.78435
      | 0.76123]
  ganshuini1 : Lookup_n-D  NumberOfTableDimensions=1  BreakpointsForDimension1=|  Table=|  InternalRulePriority=Speed  RndMeth=Simplest  InputSameDT=on
      BreakpointsForDimension1=|
      | [0
      | 0.00612
      | 0.01323
      | 0.0185
      | 0.024
      | 0.03293
      | 0.04531
      | 0.05241
      | 0.06295
      | 0.06845
      | 0.07555
      | 0.08266
      | 0.08976
      | 0.0932
      | 0.10213
      | 0.11107
      | 0.12161
      | 0.13055
      | 0.14315
      | 0.15369
      | 0.17156
      | 0.18577
      | 0.19631
      | 0.21419
      | 0.2355
      | 0.25497
      | 0.27468
      | 0.28889
      | 0.30676
      | 0.3173
      | 0.33334
      | 0.35465
      | 0.37252
      | 0.3991
      | 0.41858
      | 0.44539
      | 0.46143
      | 0.48985
      | 0.51299
      | 0.53613
      | 0.55194
      | 0.56798
      | 0.59823
      | 0.6161
      | 0.64085
      | 0.66926
      | 0.69424
      | 0.69791
      | 0.71211
      | 0.75107
      | 0.79209
      | 0.81706
      | 0.85075
      | 0.89887
      | 0.93599
      | 0.98411
      | 0.99832]
      Table=|
      | [0.0357
      | 0.13134
      | 0.30251
      | 0.41079
      | 0.52393
      | 0.63999
      | 0.78847
      | 0.84617
      | 0.90679
      | 0.9444
      | 0.97228
      | 0.99238
      | 1.01248
      | 1.02512
      | 1.04263
      | 1.05787
      | 1.06532
      | 1.07537
      | 1.07797
      | 1.08056
      | 1.08056
      | 1.07797
      | 1.07537
      | 1.06792
      | 1.05527
      | 1.05009
      | 1.04004
      | 1.03258
      | 1.02512
      | 1.01994
      | 1.00989
      | 0.99724
      | 0.98979
      | 0.97455
      | 0.9645
      | 0.94959
      | 0.94181
      | 0.92949
      | 0.91425
      | 0.90161
      | 0.89156
      | 0.8841
      | 0.86886
      | 0.86141
      | 0.84876
      | 0.82867
      | 0.81602
      | 0.81343
      | 0.80857
      | 0.78587
      | 0.76318
      | 0.75313
      | 0.73562
      | 0.70547
      | 0.69024
      | 0.66268
      | 0.6549]
  shiliqing4 : Lookup_n-D  NumberOfTableDimensions=1  BreakpointsForDimension1=|  Table=|  InternalRulePriority=Speed  RndMeth=Simplest  InputSameDT=on
      BreakpointsForDimension1=|
      | [0.00269
      | 0.00429
      | 0.01139
      | 0.01689
      | 0.02033
      | 0.0256
      | 0.0311
      | 0.04004
      | 0.04874
      | 0.06135
      | 0.07372
      | 0.08609
      | 0.0987
      | 0.11451
      | 0.13948
      | 0.1734
      | 0.20342
      | 0.23023
      | 0.24787
      | 0.26391
      | 0.28522
      | 0.30676
      | 0.3173
      | 0.35465
      | 0.39383
      | 0.42935
      | 0.47564
      | 0.51826
      | 0.55905
      | 0.59113
      | 0.63925
      | 0.68003
      | 0.72266
      | 0.7529
      | 0.79552
      | 0.84548
      | 0.89153
      | 0.92545
      | 0.99488]
      Table=|
      | [0.04835
      | 0.16927
      | 0.24707
      | 0.3278
      | 0.39328
      | 0.54662
      | 0.63221
      | 0.70547
      | 0.76059
      | 0.82607
      | 0.87405
      | 0.89901
      | 0.9243
      | 0.93694
      | 0.93954
      | 0.93694
      | 0.92689
      | 0.92171
      | 0.90906
      | 0.9042
      | 0.89415
      | 0.8841
      | 0.87665
      | 0.864
      | 0.84876
      | 0.82867
      | 0.81116
      | 0.79592
      | 0.77323
      | 0.75832
      | 0.74049
      | 0.72298
      | 0.70029
      | 0.69024
      | 0.67014
      | 0.64744
      | 0.62994
      | 0.6147
      | 0.58196]
  shiliqing5 : Lookup_n-D  NumberOfTableDimensions=1  BreakpointsForDimension1=|  Table=|  InternalRulePriority=Speed  RndMeth=Simplest  InputSameDT=on
      BreakpointsForDimension1=|
      | [8.52288E-4
      | 0.00429
      | 0.00612
      | 0.00796
      | 0.01139
      | 0.01506
      | 0.01689
      | 0.0185
      | 0.02033
      | 0.02216
      | 0.0256
      | 0.02927
      | 0.03454
      | 0.0382
      | 0.04164
      | 0.04714
      | 0.05058
      | 0.05768
      | 0.06478
      | 0.07189
      | 0.08082
      | 0.08793
      | 0.0932
      | 0.0987
      | 0.1058
      | 0.1129
      | 0.12528
      | 0.14315
      | 0.1876
      | 0.21052
      | 0.23023
      | 0.25337
      | 0.29072
      | 0.33678
      | 0.40437
      | 0.48435
      | 0.55561
      | 0.6035
      | 0.70662
      | 0.76894
      | 0.84364
      | 0.92018
      | 1.00015]
      Table=|
      | [0.04575
      | 0.09859
      | 0.14139
      | 0.19423
      | 0.24221
      | 0.285
      | 0.33525
      | 0.37059
      | 0.40074
      | 0.43348
      | 0.46622
      | 0.53171
      | 0.56672
      | 0.59201
      | 0.62475
      | 0.65231
      | 0.675
      | 0.71034
      | 0.73789
      | 0.75313
      | 0.77064
      | 0.77842
      | 0.78328
      | 0.78847
      | 0.79592
      | 0.79852
      | 0.79852
      | 0.79333
      | 0.78587
      | 0.77842
      | 0.77064
      | 0.76577
      | 0.75313
      | 0.73562
      | 0.71293
      | 0.68505
      | 0.66009
      | 0.64485
      | 0.6147
      | 0.58715
      | 0.56186
      | 0.53657
      | 0.50902]
  shiliqing6 : Lookup_n-D  NumberOfTableDimensions=1  BreakpointsForDimension1=|  Table=|  InternalRulePriority=Speed  RndMeth=Simplest  InputSameDT=on
      BreakpointsForDimension1=|
      | [0.0
      | 0.00154
      | 0.00798
      | 0.01212
      | 0.01419
      | 0.01856
      | 0.02477
      | 0.02914
      | 0.03764
      | 0.04615
      | 0.05236
      | 0.05673
      | 0.06087
      | 0.06937
      | 0.07788
      | 0.08846
      | 0.10317
      | 0.11812
      | 0.1372
      | 0.16893
      | 0.20503
      | 0.24941
      | 0.29171
      | 0.32988
      | 0.37012
      | 0.41243
      | 0.45496
      | 0.49083
      | 0.529
      | 0.57775
      | 0.62856
      | 0.68167
      | 0.73249
      | 0.77686
      | 0.82975
      | 0.90608
      | 0.94839
      | 1]
      Table=|
      | [0.0
      | 0.09756
      | 0.14551
      | 0.20878
      | 0.25379
      | 0.32
      | 0.35588
      | 0.39208
      | 0.44329
      | 0.47917
      | 0.50624
      | 0.5245
      | 0.5395
      | 0.55451
      | 0.57245
      | 0.58158
      | 0.59071
      | 0.59952
      | 0.59658
      | 0.59365
      | 0.58745
      | 0.57864
      | 0.57245
      | 0.56364
      | 0.55451
      | 0.54831
      | 0.5395
      | 0.53331
      | 0.5245
      | 0.51537
      | 0.5033
      | 0.49417
      | 0.48536
      | 0.47623
      | 0.46416
      | 0.44916
      | 0.44329
      | 0.43122]
  Out1 : Outport
  wires:
  MeaModule17/1 -> Switch/1
  PID Controller1/1 -> Saturation/1
  [S22] -> Abs1/1, Add3/1
  MeaModule1/1 -> Add3/2
  Add3/1 -> Product1/2
  Chart2/1(k1) -> Product1/1, MeaModule2/1
  MeaModule2/1 -> Switch/3, Switch/2
  Product1/1 -> PID Controller1/1
  Saturation/1 -> MeaModule17/1
  Abs1/1 -> Chart2/1(a1)
  Switch/1 -> Out1/1
  Product3/1 -> Add30/1
  Constant41/1 -> Add34/2
  Add30/1 -> Divide19/2
  Divide12/1 -> [e7]
  [e2] -> Product4/1
  [u2] -> Add33/2
  Product8/1 -> Add30/6
  Add31/1 -> Abs12/1
  Constant52/1 -> Divide13/1
  Product7/1 -> Add30/5
  [u2] -> Add35/2
  Constant1/1 -> Divide14/1
  In6/1 -> Divide6/2
  Add32/1 -> Divide20/2
  [e1] -> Product3/2
  [u2] -> Add2/2
  Divide6/1 -> [u2]
  In2/1 -> Divide6/1
  Constant13/1 -> Divide16/1
  Add19/1 -> Chart4/1(input)
  [e3] -> Add19/3
  [e5] -> Product7/1
  Chart4/1(output) -> Divide19/1
  Constant37/1 -> Add32/2
  Divide21/1 -> [e6]
  Divide19/1 -> Saturation3/1
  [e3] -> Product5/1
  Constant14/1 -> Add8/2
  [e8] -> Add19/8
  Add1/1 -> Abs11/1
  Product25/1 -> Add30/8
  Constant20/1 -> Product7/2
  Product9/1 -> Add30/7
  [e6] -> Add19/6
  shiliqing6/1 -> Add31/1
  [e8] -> Product25/1
  [e4] -> Add19/4
  shiliqing5/1 -> Add5/1
  ganliqing1/1 -> Add1/1
  Divide14/1 -> [e1]
  Constant53/1 -> Add38/2
  Divide16/1 -> [e3]
  Abs11/1 -> Add6/1
  Add2/1 -> Abs15/1
  [u2] -> Add1/2
  Constant17/1 -> Divide20/1
  Constant49/1 -> Product9/2
  Constant45/1 -> Divide12/1
  Add36/1 -> Divide12/2
  Constant18/1 -> Add6/2
  Add4/1 -> Abs13/1
  Divide20/1 -> [e5]
  Divide17/1 -> [e4]
  Product6/1 -> Add30/4
  ganshuini1/1 -> Add2/1
  [e7] -> Add19/7
  [u2] -> Add4/2
  Abs13/1 -> Add8/1
  Add34/1 -> Divide21/2
  Abs16/1 -> Add34/1
  [u2] -> Add37/2
  Constant12/1 -> Divide15/1
  Abs18/1 -> Add38/1
  Divide13/1 -> [e8]
  Constant32/1 -> Product3/1
  Abs15/1 -> Add7/1
  Abs14/1 -> Add9/1
  Add6/1 -> Divide14/2
  eluanshi4/1 -> Add35/1
  [u2] -> Add5/2
  [u2] -> Add31/2
  Abs17/1 -> Add36/1
  [e2] -> Add19/2
  [e1] -> Add19/1
  Constant15/1 -> Divide17/1
  Add5/1 -> Abs14/1
  Add8/1 -> Divide16/2
  Constant23/1 -> Add7/2
  [e6] -> Product8/1
  Add38/1 -> Divide13/2
  eluanshi3/1 -> Add33/1
  [e4] -> Product6/1
  Add37/1 -> Abs18/1
  [e5] -> Add19/5
  Add7/1 -> Divide15/2
  shiliqing4/1 -> Add4/1
  Constant16/1 -> Product6/2
  Product4/1 -> Add30/2
  Abs12/1 -> Add32/1
  Divide15/1 -> [e2]
  Constant33/1 -> Product4/2
  Constant47/1 -> Add36/2
  Constant27/1 -> Add9/2
  Constant22/1 -> Product8/2
  eluanshi5/1 -> Add37/1
  Constant21/1 -> Divide21/1
  Constant54/1 -> Product25/2
  [e7] -> Product9/1
  Product5/1 -> Add30/3
  Add35/1 -> Abs17/1
  Add33/1 -> Abs16/1
  Add9/1 -> Divide17/2
  In3/1 -> [S22], ganliqing1/1, ganshuini1/1, eluanshi4/1, eluanshi5/1, eluanshi3/1, shiliqing6/1, shiliqing5/1, shiliqing4/1
  Constant34/1 -> Product5/2
  Saturation3/1 -> MeaModule1/1
